simulink model "model4"  (R2024a)
settings: Solver=ode4  StartTime=0.0  StopTime=10.0  FixedStep=0.01  RelTol=1e-3
settings Model: Creator=TAU  LastModifiedBy=TAU

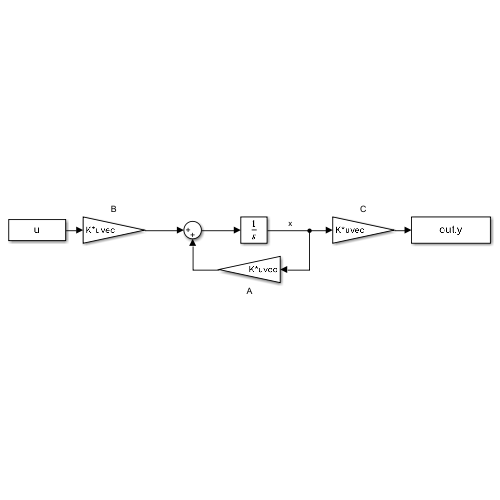
[thumbnail: Simulink's stored preview of the top-level diagram]
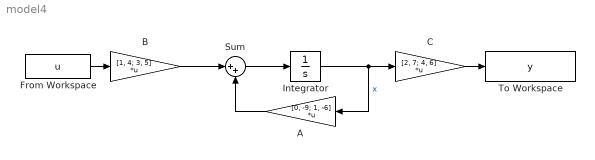
== system model4 ==
  A : Gain  Gain=[0, -9; 1, -6]  Multiplication=Matrix(K*u) (u vector)
  B : Gain  Gain=[1, 4; 3, 5]  Multiplication=Matrix(K*u) (u vector)
  C : Gain  Gain=[2, 7; 4, 6]  Multiplication=Matrix(K*u) (u vector)
  From Workspace : FromWorkspace  VariableName=u
  Integrator : Integrator
  Sum : Sum  Inputs=|++
  To Workspace : ToWorkspace  VariableName=y  SaveFormat=Timeseries  SampleTime=-1
  wires:
  A/1 -> Sum/2
  B/1 -> Sum/1
  Sum/1 -> Integrator/1
  Integrator/1 -> A/1, C/1  "x"
  C/1 -> To Workspace/1
  From Workspace/1 -> B/1
